simulink model "rotation_iterations"  (R2013a)
settings: Solver=VariableStepDiscrete  StartTime=0.0  StopTime=10  RelTol=1e-3
StopFcn:
  | % script to plot the rotations of a CORDIC engine in vectoring mode
  | % created: May 08 by Louise Crockett
  | % modified: July 08
  | %--------------------------------------------------------------------------
  | 
  | 
  | % first establish the size of the matrices holding the X and Y vectors
  | % (both X and Y are the same size)
  | % there is one row (m) for each pair of random inputs (equal to simulation length)
  | % there is one column (n) for each of the iterations
  | 
  | [m, n] = size(x_vector);
  | 
  | % if there are more than twenty samples (pairs of random inputs), restrict the
  | % treatment to the last twenty.
  | if m > 20
  |     k = m - 19;
  | else
  |     k = 1;
  | end
  | 
  | 
  | % now find vectors and plot
  | %--------------------------------------------------------------------------
  | 
  | for i = k:m-1
  | 
  |     % find the largest magnitude, so that the X and Y axes can be scaled appropriately
  |     largest_r = sqrt(x_vector(i,n)^2 + y_vector(i,n)^2);
  | 
  |     % set up vectors to draw the x axis... extend to 100% longer than the
  |     % maximum vector magnitude
  |     draw_x_axis = (0:0.01:(largest_r*2));
  |     draw_y_axis = zeros(1,length(draw_x_axis));
  | 
  |     % now, for each pair of random inputs, draw a graph of the rotation of the vector
  | 
  |     figure(i)
  |     hold off
  | 
  |     % draw the input vector (before any rotations)
  |     plot([0 x_vector(i,1)], [0 y_vector(i,1)], 'LineWidth',2);%,'m->','MarkerFaceColor','m');
  | 
  |     hold all
  | 
  |     % now draw the vector after each rotation...
  |     for j = 2:n
  |         plot([0 x_vector(i,j)], [0 y_vector(i,j)], 'LineWidth',2);%,'k->','MarkerFaceColor','k');
  |     end
  | 
  |     % draw a dotted line to connect the ends of each of the vectors
  |     plot(x_vector(i,1:end), y_vector(i,1:end),'k:');
  | 
  |     % draw the X axis (vectors should be rotated towards this
  |     plot(draw_x_axis, draw_y_axis,'k-');
  | 
  |     % set up axes scaling...
  |     axis([0 (largest_r*1.1) -largest_r largest_r]);
  |     axis square
  | 
  |     % label axes
  |     xlabel('X');
  |     ylabel('Y');
  | 
  |     % provide a title...
  |     title('Vectoring Mode Iterations');
  | 
  |     % add a legend at the right hand side
  |     % create a cell array containing the required strings
  |     legend_matrix = cell(1,n);
  |     legend_matrix(1,1) = {'Input'};
  |     for s = 2:n
  |         legend_matrix(1,s) = {['Iteration ', num2str(s-1)]};
  |     end
  |     legend(legend_matrix, 'Location', 'EastOutside');
  | 
  | end
  | 
  | 
  | % now plot the behaviour of the Z values during the iteration process
  | %-----------------------------------------------------------------------
  | 
  | marktype = ['s' 'v' '^' 'o' '>'];
  | markcolour = ['g' 'b' 'k' 'r' 'y' 'm' 'c'];
  | x_axis = [0:1:n-1];
  | 
  | figure(i+1)
  | hold off
  | plot([0 n-1],[0 0],'k:');
  | hold on
  | for j = 1:length(z_vector) - 1
  |    markcolour_index = 1+rem(j,length(markcolour));
  |    marktype_index = 1+rem(j,length(marktype));
  |    plot(x_axis,transpose(z_vector(j,1:end)),'k-','Color', markcolour(markcolour_index),'MarkerEdgeColor','k', 'MarkerFaceColor', markcolour(markcolour_index),'Marker', marktype(marktype_index));
  | end
  | xlabel('Iteration');
  | ylabel('Angle (degrees)');
  | title('Z Register');
  | 
  | % add a legend at the right hand side
  | % create a cell array containing the required strings
  | legend_matrix = cell(1,length(z_vector));
  | legend_matrix(1,1) = {'X axis'};
  | for t = 2:length(z_vector)
  |     legend_matrix(1,t) = {['Input Vector ', num2str(t-1)]};
  | end
  | legend(legend_matrix, 'Location', 'EastOutside');
libraries: xbsIndex_r4 x44
settings Model: Creator=lcrockett  LastModifiedBy=hebin
settings DataIOCC: SignalLoggingSaveFormat=ModelDataLogs  SignalLoggingName=sigsOut
settings OptimizationCC: InlineParams=on  InlineInvariantSignals=on  ExpressionDepthLimit=2147483647  InitFltsAndDblsToZero=on
settings DebuggingCC: SaveWithParameterizedLinksMsg=none  SignalResolutionControl=TryResolveAllWithWarning  SolverPrmCheckMsg=none  MultiTaskDSMMsg=warning  MultiTaskCondExecSysMsg=none  FcnCallInpInsideContextMsg=UseLocalSettings  StrictBusMsg=None
settings HardwareCC: TargetUnknown=on
settings RTWCC: IncludeERTFirstTime=on
settings GRTTargetCC: TargetFcnLib=ansi_tfl_tmw.mat  ModelReferenceCompliant=off  CombineOutputUpdateFcns=off  MatFileLogging=off  GRTInterface=on

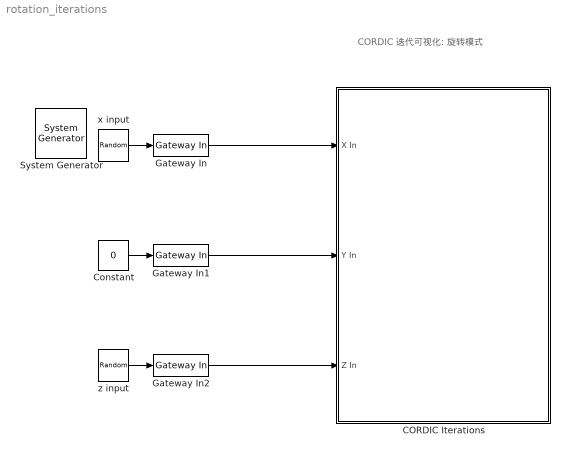
== system rotation_iterations ==
  note: CORDIC 迭代可视化: 旋转模式
  " System Generator" : xbsIndex_r4/ System Generator  Tag=genX  xilinxfamily=virtex2p  part=xc2vp30  speed=-7  package=ff896  synthesis_tool=XST  clock_wrapper=Clock Enables  directory=./netlist  proj_type=Vivado  Synth_file=Vivado Synthesis Defaults  Impl_file=Vivado Implementation Defaults  testbench=off  simulink_period=1  sysclk_period=100  dcm_input_clock_period=100  incr_netlist=off  trim_vbits=Everywhere in SubSystem  dbl_ovrd=According to Block Masks  core_generation=According to Block Masks  run_coregen=off  deprecated_control=off  eval_field=0  block_type=sysgen
      settings: block_version=8.2
  CORDIC Iterations : Subsystem
  Constant : Constant  Value=0  SampleTime=1
  Gateway In : xbsIndex_r4/Gateway In  gui_display_data_type=Fixed-point  arith_type="Signed  (2's comp)"  n_bits=15  bin_pt=12  preci_type=Single  exp_width=8  frac_width=24  quantization=Truncate  overflow=Wrap  period=1  UseAsADC=off  ADCChannel='1'  interface=None  automatic_assignment=on  address_offset=hex2dec('00')  intf_description=''  timing_constraint=None  locs_specified=off  LOCs={}  inherit_from_input=off  hdl_port=on  dbl_ovrd=off  io_standard={}  block_type=gatewayin
      settings: infoedit="Gateway in block.  Converts inputs of type Simulink integer, double and fixed point to  Xilinx fixed point type.<P><P>Hardware notes:  In hardware these blocks become top level input ports."  xl_area=[0, 0, 0, 0, 0, 0, 0]  block_version=VER_STRING_GOES_HERE
  Gateway In1 : xbsIndex_r4/Gateway In  gui_display_data_type=Fixed-point  arith_type="Signed  (2's comp)"  n_bits=15  bin_pt=12  preci_type=Single  exp_width=8  frac_width=24  quantization=Truncate  overflow=Wrap  period=1  UseAsADC=off  ADCChannel='1'  interface=None  automatic_assignment=on  address_offset=hex2dec('00')  intf_description=''  timing_constraint=None  locs_specified=off  LOCs={}  inherit_from_input=off  hdl_port=on  dbl_ovrd=off  io_standard={}  block_type=gatewayin
      settings: infoedit="Gateway in block.  Converts inputs of type Simulink integer, double and fixed point to  Xilinx fixed point type.<P><P>Hardware notes:  In hardware these blocks become top level input ports."  xl_area=[0, 0, 0, 0, 0, 0, 0]  block_version=VER_STRING_GOES_HERE
  Gateway In2 : xbsIndex_r4/Gateway In  gui_display_data_type=Fixed-point  arith_type="Signed  (2's comp)"  n_bits=19  bin_pt=12  preci_type=Single  exp_width=8  frac_width=24  quantization=Truncate  overflow=Wrap  period=1  UseAsADC=off  ADCChannel='1'  interface=None  automatic_assignment=on  address_offset=hex2dec('00')  intf_description=''  timing_constraint=None  locs_specified=off  LOCs={}  inherit_from_input=off  hdl_port=on  dbl_ovrd=off  io_standard={}  block_type=gatewayin
      settings: infoedit="Gateway in block.  Converts inputs of type Simulink integer, double and fixed point to  Xilinx fixed point type.<P><P>Hardware notes:  In hardware these blocks become top level input ports."  xl_area=[0, 0, 0, 0, 0, 0, 0]  block_version=VER_STRING_GOES_HERE
  x input : UniformRandomNumber  Minimum=0  Maximum=0.5  Seed=579  SampleTime=1
  z input : UniformRandomNumber  Minimum=-90  Maximum=90  Seed=106  SampleTime=1
  wires:
  x input/1 -> Gateway In/1
  Constant/1 -> Gateway In1/1
  Gateway In/1 -> CORDIC Iterations/1(X In)
  Gateway In1/1 -> CORDIC Iterations/2(Y In)
  z input/1 -> Gateway In2/1
  Gateway In2/1 -> CORDIC Iterations/3(Z In)

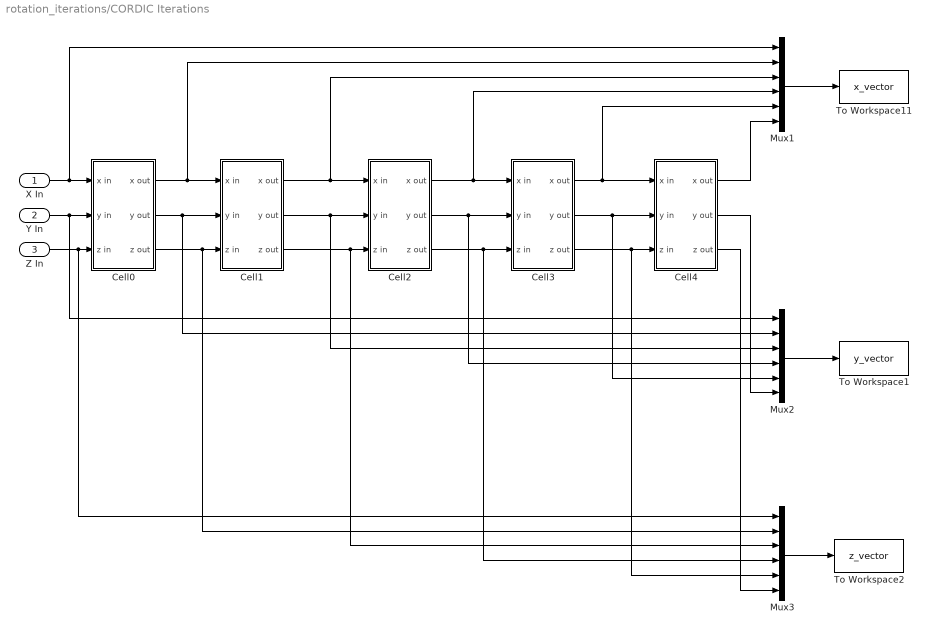
== system rotation_iterations/CORDIC Iterations ==
  X In : Inport
  Y In : Inport  Port=2
  Z In : Inport  Port=3
  Cell0 : Subsystem
  Cell1 : Subsystem
  Cell2 : Subsystem
  Cell3 : Subsystem
  Cell4 : Subsystem
  Mux1 : Mux  Inputs=6
  Mux2 : Mux  Inputs=6
  Mux3 : Mux  Inputs=6
  To Workspace1 : ToWorkspace  VariableName=y_vector  SampleTime=-1
  To Workspace11 : ToWorkspace  VariableName=x_vector  SampleTime=-1
  To Workspace2 : ToWorkspace  VariableName=z_vector  SampleTime=-1
  wires:
  X In/1 -> Mux1/1, Cell0/1(x in)
  Y In/1 -> Mux2/1, Cell0/2(y in)
  Cell0/1(x out) -> Mux1/2, Cell1/1(x in)
  Cell0/2(y out) -> Mux2/2, Cell1/2(y in)
  Cell1/1(x out) -> Mux1/3, Cell2/1(x in)
  Cell1/2(y out) -> Mux2/3, Cell2/2(y in)
  Cell2/1(x out) -> Mux1/4, Cell3/1(x in)
  Cell2/2(y out) -> Mux2/4, Cell3/2(y in)
  Cell3/1(x out) -> Mux1/5, Cell4/1(x in)
  Cell3/2(y out) -> Mux2/5, Cell4/2(y in)
  Cell4/1(x out) -> Mux1/6
  Mux1/1 -> To Workspace11/1
  Mux2/1 -> To Workspace1/1
  Cell4/2(y out) -> Mux2/6
  Z In/1 -> Cell0/3(z in), Mux3/1
  Cell0/3(z out) -> Cell1/3(z in), Mux3/2
  Cell1/3(z out) -> Cell2/3(z in), Mux3/3
  Cell2/3(z out) -> Cell3/3(z in), Mux3/4
  Cell3/3(z out) -> Cell4/3(z in), Mux3/5
  Mux3/1 -> To Workspace2/1
  Cell4/3(z out) -> Mux3/6

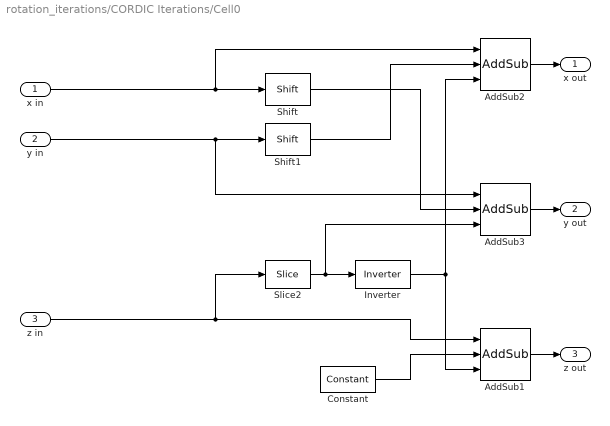
== system rotation_iterations/CORDIC Iterations/Cell0 ==
  x in : Inport
  y in : Inport  Port=2
  z in : Inport  Port=3
  AddSub1 : xbsIndex_r4/AddSub  mode=Addition or Subtraction  use_carryin=off  use_carryout=off  en=off  latency=0  precision=User Defined  arith_type="Signed  (2's comp)"  n_bits=20  bin_pt=12  quantization=Truncate  overflow=Wrap  use_behavioral_HDL=on  hw_selection=Fabric  pipelined=off  use_rpm=on  dbl_ovrd=off  block_type=addsub
      settings: xl_area=[0, 0, 0, 0, 0, 0, 0]  block_version=VER_STRING_GOES_HERE
  AddSub2 : xbsIndex_r4/AddSub  mode=Addition or Subtraction  use_carryin=off  use_carryout=off  en=off  latency=0  precision=User Defined  arith_type="Signed  (2's comp)"  n_bits=15  bin_pt=12  quantization=Truncate  overflow=Wrap  use_behavioral_HDL=on  hw_selection=Fabric  pipelined=off  use_rpm=on  dbl_ovrd=off  block_type=addsub
      settings: xl_area=[0, 0, 0, 0, 0, 0, 0]  block_version=VER_STRING_GOES_HERE
  AddSub3 : xbsIndex_r4/AddSub  mode=Addition or Subtraction  use_carryin=off  use_carryout=off  en=off  latency=0  precision=User Defined  arith_type="Signed  (2's comp)"  n_bits=15  bin_pt=12  quantization=Truncate  overflow=Wrap  use_behavioral_HDL=on  hw_selection=Fabric  pipelined=off  use_rpm=on  dbl_ovrd=off  block_type=addsub
      settings: xl_area=[0, 0, 0, 0, 0, 0, 0]  block_version=VER_STRING_GOES_HERE
  Constant : xbsIndex_r4/Constant  const=45  gui_display_data_type=Fixed-point  arith_type=Signed (2's comp)  n_bits=20  bin_pt=12  preci_type=Single  exp_width=8  frac_width=24  explicit_period=off  period=1  equ=P=C  opselect=C  inp2=PCIN>>17  opr=+  inp1=P  carry=CIN  dbl_ovrd=off  block_type=constant
      settings: block_version=10.1.2
  Inverter : xbsIndex_r4/Inverter  en=off  latency=0  dbl_ovrd=off  block_type=inv
      settings: block_version=10.1.2
  Shift : xbsIndex_r4/Shift  shift_dir=Right  shift_bits=0  en=off  latency=0  precision=User Defined  arith_type="Signed  (2's comp)"  n_bits=15  bin_pt=12  quantization=Truncate  overflow=Wrap  dbl_ovrd=off  block_type=shift
      settings: xl_area=[0, 0, 0, 0, 0, 0, 0]  block_version=VER_STRING_GOES_HERE
  Shift1 : xbsIndex_r4/Shift  shift_dir=Right  shift_bits=0  en=off  latency=0  precision=User Defined  arith_type="Signed  (2's comp)"  n_bits=15  bin_pt=12  quantization=Truncate  overflow=Wrap  dbl_ovrd=off  block_type=shift
      settings: xl_area=[0, 0, 0, 0, 0, 0, 0]  block_version=VER_STRING_GOES_HERE
  Slice2 : xbsIndex_r4/Slice  nbits=1  boolean_output=on  mode=Upper Bit Location + Width  bit1=0  base1=MSB of Input  bit0=0  base0=LSB of Input  dbl_ovrd=off  block_type=slice
      settings: infoedit="Extracts a given range of bits from each input sample and presents it at the output.  The output type is ordinarily unsigned with binary point at zero, but can be Boolean when the slice is one bit wide.<P><P>Hardware notes: In hardware this block costs nothing."  block_version=VER_STRING_GOES_HERE
  x out : Outport
  y out : Outport  Port=2
  z out : Outport  Port=3
  wires:
  x in/1 -> AddSub2/1, Shift/1
  y in/1 -> AddSub3/1, Shift1/1
  Shift1/1 -> AddSub2/2
  Shift/1 -> AddSub3/2
  AddSub2/1 -> x out/1
  AddSub3/1 -> y out/1
  z in/1 -> AddSub1/1, Slice2/1
  Constant/1 -> AddSub1/2
  Slice2/1 -> Inverter/1, AddSub3/3
  AddSub1/1 -> z out/1
  Inverter/1 -> AddSub1/3, AddSub2/3

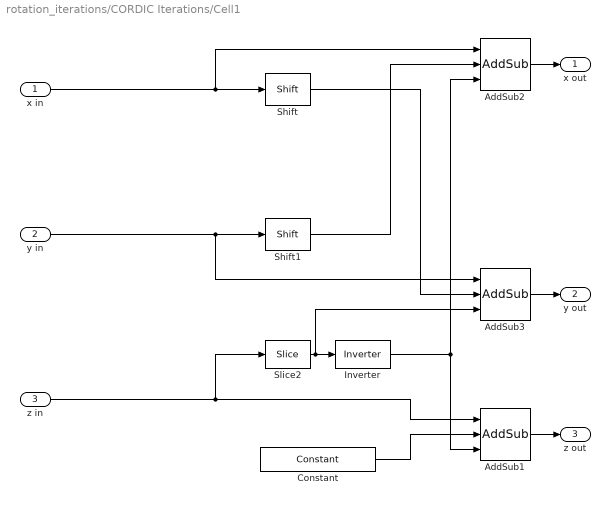
== system rotation_iterations/CORDIC Iterations/Cell1 ==
  x in : Inport
  y in : Inport  Port=2
  z in : Inport  Port=3
  AddSub1 : xbsIndex_r4/AddSub  mode=Addition or Subtraction  use_carryin=off  use_carryout=off  en=off  latency=0  precision=User Defined  arith_type="Signed  (2's comp)"  n_bits=20  bin_pt=12  quantization=Truncate  overflow=Wrap  use_behavioral_HDL=on  hw_selection=Fabric  pipelined=off  use_rpm=on  dbl_ovrd=off  block_type=addsub
      settings: xl_area=[0, 0, 0, 0, 0, 0, 0]  block_version=VER_STRING_GOES_HERE
  AddSub2 : xbsIndex_r4/AddSub  mode=Addition or Subtraction  use_carryin=off  use_carryout=off  en=off  latency=0  precision=User Defined  arith_type="Signed  (2's comp)"  n_bits=15  bin_pt=12  quantization=Truncate  overflow=Wrap  use_behavioral_HDL=on  hw_selection=Fabric  pipelined=off  use_rpm=on  dbl_ovrd=off  block_type=addsub
      settings: xl_area=[0, 0, 0, 0, 0, 0, 0]  block_version=VER_STRING_GOES_HERE
  AddSub3 : xbsIndex_r4/AddSub  mode=Addition or Subtraction  use_carryin=off  use_carryout=off  en=off  latency=0  precision=User Defined  arith_type="Signed  (2's comp)"  n_bits=15  bin_pt=12  quantization=Truncate  overflow=Wrap  use_behavioral_HDL=on  hw_selection=Fabric  pipelined=off  use_rpm=on  dbl_ovrd=off  block_type=addsub
      settings: xl_area=[0, 0, 0, 0, 0, 0, 0]  block_version=VER_STRING_GOES_HERE
  Constant : xbsIndex_r4/Constant  const=26.5650511771  gui_display_data_type=Fixed-point  arith_type=Signed (2's comp)  n_bits=20  bin_pt=12  preci_type=Single  exp_width=8  frac_width=24  explicit_period=off  period=1  equ=P=C  opselect=C  inp2=PCIN>>17  opr=+  inp1=P  carry=CIN  dbl_ovrd=off  block_type=constant
      settings: block_version=10.1.2
  Inverter : xbsIndex_r4/Inverter  en=off  latency=0  dbl_ovrd=off  block_type=inv
      settings: block_version=10.1.2
  Shift : xbsIndex_r4/Shift  shift_dir=Right  shift_bits=1  en=off  latency=0  precision=User Defined  arith_type="Signed  (2's comp)"  n_bits=15  bin_pt=12  quantization=Truncate  overflow=Wrap  dbl_ovrd=off  block_type=shift
      settings: xl_area=[0, 0, 0, 0, 0, 0, 0]  block_version=VER_STRING_GOES_HERE
  Shift1 : xbsIndex_r4/Shift  shift_dir=Right  shift_bits=1  en=off  latency=0  precision=User Defined  arith_type="Signed  (2's comp)"  n_bits=15  bin_pt=12  quantization=Truncate  overflow=Wrap  dbl_ovrd=off  block_type=shift
      settings: xl_area=[0, 0, 0, 0, 0, 0, 0]  block_version=VER_STRING_GOES_HERE
  Slice2 : xbsIndex_r4/Slice  nbits=1  boolean_output=on  mode=Upper Bit Location + Width  bit1=0  base1=MSB of Input  bit0=0  base0=LSB of Input  dbl_ovrd=off  block_type=slice
      settings: infoedit="Extracts a given range of bits from each input sample and presents it at the output.  The output type is ordinarily unsigned with binary point at zero, but can be Boolean when the slice is one bit wide.<P><P>Hardware notes: In hardware this block costs nothing."  block_version=VER_STRING_GOES_HERE
  x out : Outport
  y out : Outport  Port=2
  z out : Outport  Port=3
  wires:
  x in/1 -> AddSub2/1, Shift/1
  y in/1 -> AddSub3/1, Shift1/1
  Shift1/1 -> AddSub2/2
  Shift/1 -> AddSub3/2
  AddSub2/1 -> x out/1
  AddSub3/1 -> y out/1
  z in/1 -> AddSub1/1, Slice2/1
  Constant/1 -> AddSub1/2
  AddSub1/1 -> z out/1
  Slice2/1 -> Inverter/1, AddSub3/3
  Inverter/1 -> AddSub1/3, AddSub2/3

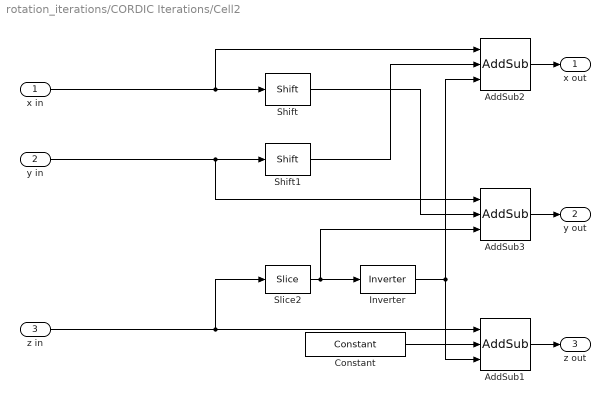
== system rotation_iterations/CORDIC Iterations/Cell2 ==
  x in : Inport
  y in : Inport  Port=2
  z in : Inport  Port=3
  AddSub1 : xbsIndex_r4/AddSub  mode=Addition or Subtraction  use_carryin=off  use_carryout=off  en=off  latency=0  precision=User Defined  arith_type="Signed  (2's comp)"  n_bits=20  bin_pt=12  quantization=Truncate  overflow=Wrap  use_behavioral_HDL=on  hw_selection=Fabric  pipelined=off  use_rpm=on  dbl_ovrd=off  block_type=addsub
      settings: xl_area=[0, 0, 0, 0, 0, 0, 0]  block_version=VER_STRING_GOES_HERE
  AddSub2 : xbsIndex_r4/AddSub  mode=Addition or Subtraction  use_carryin=off  use_carryout=off  en=off  latency=0  precision=User Defined  arith_type="Signed  (2's comp)"  n_bits=15  bin_pt=12  quantization=Truncate  overflow=Wrap  use_behavioral_HDL=on  hw_selection=Fabric  pipelined=off  use_rpm=on  dbl_ovrd=off  block_type=addsub
      settings: xl_area=[0, 0, 0, 0, 0, 0, 0]  block_version=VER_STRING_GOES_HERE
  AddSub3 : xbsIndex_r4/AddSub  mode=Addition or Subtraction  use_carryin=off  use_carryout=off  en=off  latency=0  precision=User Defined  arith_type="Signed  (2's comp)"  n_bits=15  bin_pt=12  quantization=Truncate  overflow=Wrap  use_behavioral_HDL=on  hw_selection=Fabric  pipelined=off  use_rpm=on  dbl_ovrd=off  block_type=addsub
      settings: xl_area=[0, 0, 0, 0, 0, 0, 0]  block_version=VER_STRING_GOES_HERE
  Constant : xbsIndex_r4/Constant  const=14.0362434679  gui_display_data_type=Fixed-point  arith_type=Signed (2's comp)  n_bits=20  bin_pt=12  preci_type=Single  exp_width=8  frac_width=24  explicit_period=off  period=1  equ=P=C  opselect=C  inp2=PCIN>>17  opr=+  inp1=P  carry=CIN  dbl_ovrd=off  block_type=constant
      settings: block_version=10.1.2
  Inverter : xbsIndex_r4/Inverter  en=off  latency=0  dbl_ovrd=off  block_type=inv
      settings: block_version=10.1.2
  Shift : xbsIndex_r4/Shift  shift_dir=Right  shift_bits=2  en=off  latency=0  precision=User Defined  arith_type="Signed  (2's comp)"  n_bits=15  bin_pt=12  quantization=Truncate  overflow=Wrap  dbl_ovrd=off  block_type=shift
      settings: xl_area=[0, 0, 0, 0, 0, 0, 0]  block_version=VER_STRING_GOES_HERE
  Shift1 : xbsIndex_r4/Shift  shift_dir=Right  shift_bits=2  en=off  latency=0  precision=User Defined  arith_type="Signed  (2's comp)"  n_bits=15  bin_pt=12  quantization=Truncate  overflow=Wrap  dbl_ovrd=off  block_type=shift
      settings: xl_area=[0, 0, 0, 0, 0, 0, 0]  block_version=VER_STRING_GOES_HERE
  Slice2 : xbsIndex_r4/Slice  nbits=1  boolean_output=on  mode=Upper Bit Location + Width  bit1=0  base1=MSB of Input  bit0=0  base0=LSB of Input  dbl_ovrd=off  block_type=slice
      settings: infoedit="Extracts a given range of bits from each input sample and presents it at the output.  The output type is ordinarily unsigned with binary point at zero, but can be Boolean when the slice is one bit wide.<P><P>Hardware notes: In hardware this block costs nothing."  block_version=VER_STRING_GOES_HERE
  x out : Outport
  y out : Outport  Port=2
  z out : Outport  Port=3
  wires:
  x in/1 -> AddSub2/1, Shift/1
  y in/1 -> AddSub3/1, Shift1/1
  Shift1/1 -> AddSub2/2
  Shift/1 -> AddSub3/2
  AddSub2/1 -> x out/1
  AddSub3/1 -> y out/1
  z in/1 -> AddSub1/1, Slice2/1
  Constant/1 -> AddSub1/2
  Slice2/1 -> Inverter/1, AddSub3/3
  AddSub1/1 -> z out/1
  Inverter/1 -> AddSub1/3, AddSub2/3

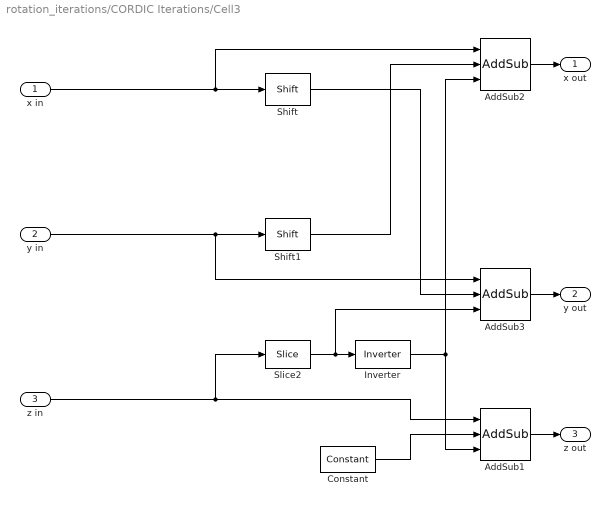
== system rotation_iterations/CORDIC Iterations/Cell3 ==
  x in : Inport
  y in : Inport  Port=2
  z in : Inport  Port=3
  AddSub1 : xbsIndex_r4/AddSub  mode=Addition or Subtraction  use_carryin=off  use_carryout=off  en=off  latency=0  precision=User Defined  arith_type="Signed  (2's comp)"  n_bits=20  bin_pt=12  quantization=Truncate  overflow=Wrap  use_behavioral_HDL=on  hw_selection=Fabric  pipelined=off  use_rpm=on  dbl_ovrd=off  block_type=addsub
      settings: xl_area=[0, 0, 0, 0, 0, 0, 0]  block_version=VER_STRING_GOES_HERE
  AddSub2 : xbsIndex_r4/AddSub  mode=Addition or Subtraction  use_carryin=off  use_carryout=off  en=off  latency=0  precision=User Defined  arith_type="Signed  (2's comp)"  n_bits=15  bin_pt=12  quantization=Truncate  overflow=Wrap  use_behavioral_HDL=on  hw_selection=Fabric  pipelined=off  use_rpm=on  dbl_ovrd=off  block_type=addsub
      settings: xl_area=[0, 0, 0, 0, 0, 0, 0]  block_version=VER_STRING_GOES_HERE
  AddSub3 : xbsIndex_r4/AddSub  mode=Addition or Subtraction  use_carryin=off  use_carryout=off  en=off  latency=0  precision=User Defined  arith_type="Signed  (2's comp)"  n_bits=15  bin_pt=12  quantization=Truncate  overflow=Wrap  use_behavioral_HDL=on  hw_selection=Fabric  pipelined=off  use_rpm=on  dbl_ovrd=off  block_type=addsub
      settings: xl_area=[0, 0, 0, 0, 0, 0, 0]  block_version=VER_STRING_GOES_HERE
  Constant : xbsIndex_r4/Constant  const=7.1250163489  gui_display_data_type=Fixed-point  arith_type=Signed (2's comp)  n_bits=20  bin_pt=12  preci_type=Single  exp_width=8  frac_width=24  explicit_period=off  period=1  equ=P=C  opselect=C  inp2=PCIN>>17  opr=+  inp1=P  carry=CIN  dbl_ovrd=off  block_type=constant
      settings: block_version=10.1.2
  Inverter : xbsIndex_r4/Inverter  en=off  latency=0  dbl_ovrd=off  block_type=inv
      settings: block_version=10.1.2
  Shift : xbsIndex_r4/Shift  shift_dir=Right  shift_bits=3  en=off  latency=0  precision=User Defined  arith_type="Signed  (2's comp)"  n_bits=15  bin_pt=12  quantization=Truncate  overflow=Wrap  dbl_ovrd=off  block_type=shift
      settings: xl_area=[0, 0, 0, 0, 0, 0, 0]  block_version=VER_STRING_GOES_HERE
  Shift1 : xbsIndex_r4/Shift  shift_dir=Right  shift_bits=3  en=off  latency=0  precision=User Defined  arith_type="Signed  (2's comp)"  n_bits=15  bin_pt=12  quantization=Truncate  overflow=Wrap  dbl_ovrd=off  block_type=shift
      settings: xl_area=[0, 0, 0, 0, 0, 0, 0]  block_version=VER_STRING_GOES_HERE
  Slice2 : xbsIndex_r4/Slice  nbits=1  boolean_output=on  mode=Upper Bit Location + Width  bit1=0  base1=MSB of Input  bit0=0  base0=LSB of Input  dbl_ovrd=off  block_type=slice
      settings: infoedit="Extracts a given range of bits from each input sample and presents it at the output.  The output type is ordinarily unsigned with binary point at zero, but can be Boolean when the slice is one bit wide.<P><P>Hardware notes: In hardware this block costs nothing."  block_version=VER_STRING_GOES_HERE
  x out : Outport
  y out : Outport  Port=2
  z out : Outport  Port=3
  wires:
  x in/1 -> AddSub2/1, Shift/1
  y in/1 -> AddSub3/1, Shift1/1
  Shift1/1 -> AddSub2/2
  Shift/1 -> AddSub3/2
  AddSub2/1 -> x out/1
  AddSub3/1 -> y out/1
  z in/1 -> AddSub1/1, Slice2/1
  Constant/1 -> AddSub1/2
  Slice2/1 -> Inverter/1, AddSub3/3
  AddSub1/1 -> z out/1
  Inverter/1 -> AddSub1/3, AddSub2/3

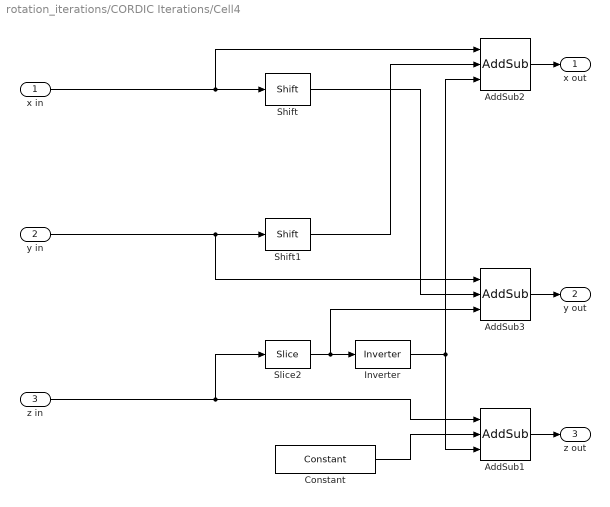
== system rotation_iterations/CORDIC Iterations/Cell4 ==
  x in : Inport
  y in : Inport  Port=2
  z in : Inport  Port=3
  AddSub1 : xbsIndex_r4/AddSub  mode=Addition or Subtraction  use_carryin=off  use_carryout=off  en=off  latency=0  precision=User Defined  arith_type="Signed  (2's comp)"  n_bits=20  bin_pt=12  quantization=Truncate  overflow=Wrap  use_behavioral_HDL=on  hw_selection=Fabric  pipelined=off  use_rpm=on  dbl_ovrd=off  block_type=addsub
      settings: xl_area=[0, 0, 0, 0, 0, 0, 0]  block_version=VER_STRING_GOES_HERE
  AddSub2 : xbsIndex_r4/AddSub  mode=Addition or Subtraction  use_carryin=off  use_carryout=off  en=off  latency=0  precision=User Defined  arith_type="Signed  (2's comp)"  n_bits=15  bin_pt=12  quantization=Truncate  overflow=Wrap  use_behavioral_HDL=on  hw_selection=Fabric  pipelined=off  use_rpm=on  dbl_ovrd=off  block_type=addsub
      settings: xl_area=[0, 0, 0, 0, 0, 0, 0]  block_version=VER_STRING_GOES_HERE
  AddSub3 : xbsIndex_r4/AddSub  mode=Addition or Subtraction  use_carryin=off  use_carryout=off  en=off  latency=0  precision=User Defined  arith_type="Signed  (2's comp)"  n_bits=15  bin_pt=12  quantization=Truncate  overflow=Wrap  use_behavioral_HDL=on  hw_selection=Fabric  pipelined=off  use_rpm=on  dbl_ovrd=off  block_type=addsub
      settings: xl_area=[0, 0, 0, 0, 0, 0, 0]  block_version=VER_STRING_GOES_HERE
  Constant : xbsIndex_r4/Constant  const=3.5763343750  gui_display_data_type=Fixed-point  arith_type=Signed (2's comp)  n_bits=20  bin_pt=12  preci_type=Single  exp_width=8  frac_width=24  explicit_period=off  period=1  equ=P=C  opselect=C  inp2=PCIN>>17  opr=+  inp1=P  carry=CIN  dbl_ovrd=off  block_type=constant
      settings: block_version=10.1.2
  Inverter : xbsIndex_r4/Inverter  en=off  latency=0  dbl_ovrd=off  block_type=inv
      settings: block_version=10.1.2
  Shift : xbsIndex_r4/Shift  shift_dir=Right  shift_bits=4  en=off  latency=0  precision=User Defined  arith_type="Signed  (2's comp)"  n_bits=15  bin_pt=12  quantization=Truncate  overflow=Wrap  dbl_ovrd=off  block_type=shift
      settings: xl_area=[0, 0, 0, 0, 0, 0, 0]  block_version=VER_STRING_GOES_HERE
  Shift1 : xbsIndex_r4/Shift  shift_dir=Right  shift_bits=4  en=off  latency=0  precision=User Defined  arith_type="Signed  (2's comp)"  n_bits=15  bin_pt=12  quantization=Truncate  overflow=Wrap  dbl_ovrd=off  block_type=shift
      settings: xl_area=[0, 0, 0, 0, 0, 0, 0]  block_version=VER_STRING_GOES_HERE
  Slice2 : xbsIndex_r4/Slice  nbits=1  boolean_output=on  mode=Upper Bit Location + Width  bit1=0  base1=MSB of Input  bit0=0  base0=LSB of Input  dbl_ovrd=off  block_type=slice
      settings: infoedit="Extracts a given range of bits from each input sample and presents it at the output.  The output type is ordinarily unsigned with binary point at zero, but can be Boolean when the slice is one bit wide.<P><P>Hardware notes: In hardware this block costs nothing."  block_version=VER_STRING_GOES_HERE
  x out : Outport
  y out : Outport  Port=2
  z out : Outport  Port=3
  wires:
  x in/1 -> AddSub2/1, Shift/1
  y in/1 -> AddSub3/1, Shift1/1
  Shift1/1 -> AddSub2/2
  Shift/1 -> AddSub3/2
  AddSub2/1 -> x out/1
  AddSub3/1 -> y out/1
  z in/1 -> AddSub1/1, Slice2/1
  Constant/1 -> AddSub1/2
  Slice2/1 -> Inverter/1, AddSub3/3
  AddSub1/1 -> z out/1
  Inverter/1 -> AddSub1/3, AddSub2/3
